simulink model "sbd"  (Simulink 6.6)
settings: Solver=FixedStepDiscrete  StartTime=0.0  StopTime=99999  RelTol=1e-3
undefined symbols (not defined in the file): gray, Rec, SDTV
libraries: simulink x5, vipsnks x3, vipstatistics x2, viptextngfix x2, vipconversions x2, dspwin32 x1, dspsnks4 x1
settings Model: Creator=leszczuk  LastModifiedBy=leszczuk
settings DebuggingCC: SolverPrmCheckMsg=none  ParameterPrecisionLossMsg=none

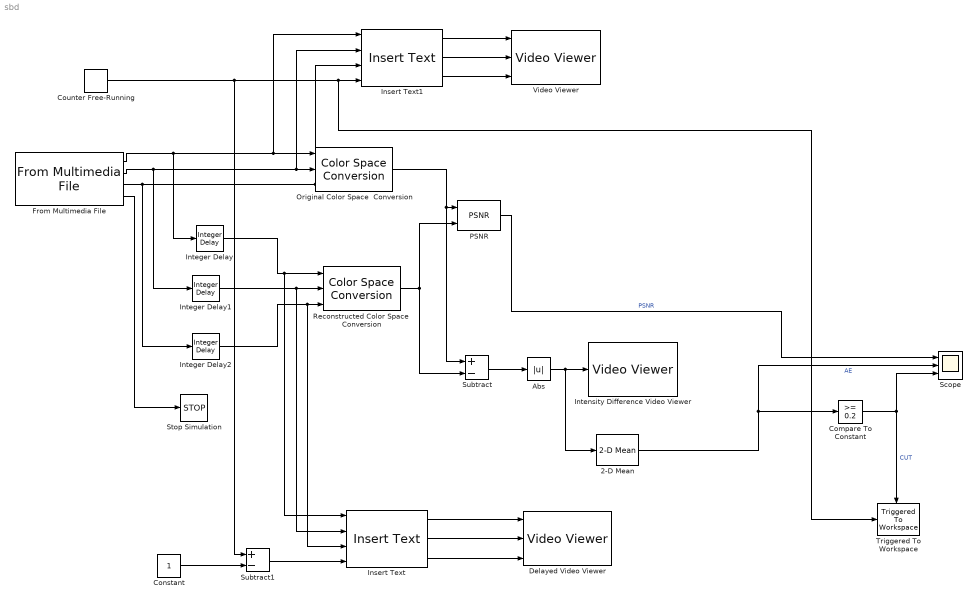
== system sbd ==
  2-D Mean : vipstatistics/2-D Mean  DialogController=vipDDGCreate  DialogControllerArgs=DataTag0  run=off  reset_popup=None  roiEnable=off  roiType=Rectangles  roiPortion=Entire ROI  roiOutput=Individual statistics for each ROI  roiFlag=off  roundingMode=Floor  overflowMode=off
  Abs : Abs
  Compare To Constant : simulink/Logic and Bit Operations/Compare To Constant  SystemSampleTime=-1  relop=>=  const=0.2  LogicOutDataTypeMode=uint8  ZeroCross=off
  Constant : Constant
  Counter Free-Running : simulink/Sources/Counter Free-Running  SystemSampleTime=-1  NumBits=16  tsamp=-1
  Delayed Video Viewer : vipsnks/Video Viewer  DialogController=vipDDGCreate  DialogControllerArgs=DataTag1  inputType=Obsolete  imagePorts=Separate color signals  useColorMap=off  colormapValue=gray(256)  specRange=off  minInputVal=0  maxInputVal=255  FigPos=[43 391 454 294]  AxisZoom=off  trueSizedOnce=on
  From Multimedia File : dspwin32/From Multimedia File  DialogController=dspDDGCreate  DialogControllerArgs=DataTag2  inputFilename=C:\Documents and Settings\leszczuk\My Documents\Dydaktyka\exercises\sbd\technologie_i_narzedzia_realizacji_systemow_multimedialnych_-_detekcja_granic_ujec\UGS05.mpg  loop=on  numPlays=1  outputStreams=Video only  videoDataType=single  audioDataType=int16  inheritSampleTime=on  userDefinedSampleTime=1/30  noAudioOutput=off  isIntensityVideo=off  colorVideoFormat=Separate color signals  outputEOF=on  dataOrg=Column-major
  Insert Text : viptextngfix/Insert Text  inputType=Obsolete  theText='preFNum=%d'  fontFace=LucidaSansRegular  dummyVar1=0  blockFontSize=36  antiAliased=on  getTextLocFrom=Specify via dialog  textLoc=[0 0]  getTextColorFrom=Specify via dialog  textColor=[255 255 0]  getTextIntensityFrom=Specify via dialog  textIntensity=0  getTextOpacityFrom=Specify via dialog  textOpacity=1.0  dummyVar2=0  dummyVar3=0  dummyVar4=0  imagePorts=Separate color signals
  Insert Text1 : viptextngfix/Insert Text  inputType=Obsolete  theText='postFNum=%d'  fontFace=LucidaSansRegular  dummyVar1=0  blockFontSize=36  antiAliased=on  getTextLocFrom=Specify via dialog  textLoc=[0 0]  getTextColorFrom=Specify via dialog  textColor=[255 255 0]  getTextIntensityFrom=Specify via dialog  textIntensity=0  getTextOpacityFrom=Specify via dialog  textOpacity=1.0  dummyVar2=0  dummyVar3=0  dummyVar4=0  imagePorts=Separate color signals
  Integer Delay : simulink/Discrete/Integer Delay  vinit=0.0  samptime=-1  NumDelays=1
  Integer Delay1 : simulink/Discrete/Integer Delay  vinit=0.0  samptime=-1  NumDelays=1
  Integer Delay2 : simulink/Discrete/Integer Delay  vinit=0.0  samptime=-1  NumDelays=1
  Intensity Difference Video Viewer : vipsnks/Video Viewer  DialogController=vipDDGCreate  DialogControllerArgs=DataTag3  inputType=Obsolete  imagePorts=One multidimensional signal  useColorMap=off  colormapValue=gray(256)  specRange=off  minInputVal=0  maxInputVal=255  FigPos=[395 41 454 294]  AxisZoom=off  trueSizedOnce=on
  Original Color Space  Conversion : vipconversions/Color Space  Conversion  conversion=Obsolete  conversionActive=R'G'B' to intensity  wp_str=D65  rec=Rec. 601 (SDTV)  sys=1125/60/2:1  imagePorts=Separate color signals
  PSNR : vipstatistics/PSNR
  Reconstructed Color Space  Conversion : vipconversions/Color Space  Conversion  conversion=Obsolete  conversionActive=R'G'B' to intensity  wp_str=D65  rec=Rec. 601 (SDTV)  sys=1125/60/2:1  imagePorts=Separate color signals
  Scope : Scope  NumInputPorts=3
      settings: TimeRange=59.9815  YMin=5~0~0  YMax=55~0.425~1
  Stop Simulation : Stop
  Subtract : Sum  Inputs=+-  OutScaling=2^-10
  Subtract1 : Sum  Inputs=+-  OutDataTypeMode=int16  OutScaling=2^-10
  Triggered To Workspace : dspsnks4/Triggered To Workspace  SystemSampleTime=-1  TriggerType=Rising edge  VariableName=autoPostFNum  Buffer=1000
      settings: FixptAsFi=off
  Video Viewer : vipsnks/Video Viewer  DialogController=vipDDGCreate  DialogControllerArgs=DataTag4  inputType=Obsolete  imagePorts=Separate color signals  useColorMap=off  colormapValue=gray(256)  specRange=off  minInputVal=0  maxInputVal=255  FigPos=[767 397 454 294]  AxisZoom=off  trueSizedOnce=on
  wires:
  PSNR/1 -> Scope/1  "PSNR"
  From Multimedia File/1 -> Integer Delay/1, Original Color Space  Conversion/1, Insert Text1/1
  Original Color Space  Conversion/1 -> Subtract/1, PSNR/1
  Reconstructed Color Space  Conversion/1 -> PSNR/2, Subtract/2
  From Multimedia File/2 -> Integer Delay1/1, Original Color Space  Conversion/2, Insert Text1/2
  From Multimedia File/3 -> Integer Delay2/1, Original Color Space  Conversion/3, Insert Text1/3
  Integer Delay1/1 -> Reconstructed Color Space  Conversion/2, Insert Text/2
  2-D Mean/1 -> Scope/2, Compare To Constant/1  "AE"
  Subtract/1 -> Abs/1
  Abs/1 -> Intensity Difference Video Viewer/1, 2-D Mean/1
  Integer Delay2/1 -> Reconstructed Color Space  Conversion/3, Insert Text/3
  Integer Delay/1 -> Reconstructed Color Space  Conversion/1, Insert Text/1
  Insert Text/1 -> Delayed Video Viewer/1
  Insert Text/2 -> Delayed Video Viewer/2
  Insert Text/3 -> Delayed Video Viewer/3
  Insert Text1/1 -> Video Viewer/1
  Insert Text1/2 -> Video Viewer/2
  Insert Text1/3 -> Video Viewer/3
  Counter Free-Running/1 -> Subtract1/1, Insert Text1/4, Triggered To Workspace/1
  Subtract1/1 -> Insert Text/4
  Constant/1 -> Subtract1/2
  Compare To Constant/1 -> Scope/3, Triggered To Workspace/Trigger  "CUT"
  From Multimedia File/4 -> Stop Simulation/1
